simulink model "Full_load_sim_doc"  (R2020a)
settings: Solver=VariableStepAuto  StartTime=0.0  StopTime=50000  RelTol=1e-3
values from neighbouring files (symbols this model uses):
  BlySyreON = 1    [sim_starter.m]
  LiIonLilleON = 1    [sim_starter.m]
  LiIonStorON = 1    [sim_starter.m]
  LoadBlySyre = load    [sim_starter.m]
  LoadLille = load    [sim_starter.m]
  LoadLiStor = 0    [sim_starter.m]
  LoadNiMH = load    [sim_starter.m]
  LoadSaltVand = load    [sim_starter.m]
  NiMHON = 1    [sim_starter.m]
  SaltVandON = 1    [sim_starter.m]
undefined symbols (not defined in the file or in its folder): Hydride, Metal, Nickel
libraries: nesl_utility x28, fl_lib x24, powerlib x4, ee_lib x4, electricdrivelib x1
(part 2 of 2)

== system Full_load_sim_doc/Afladning/LoadSaltvandCircuit ==
  CutOff : Inport
  current : Inport  Port=2
  Constant1 : Constant  Value=0
  Controlled Current Source : fl_lib/Electrical/Electrical Sources/Controlled Current Source
  Electrical Reference1 : fl_lib/Electrical/Electrical Elements/Electrical Reference
  Gain : Gain
  Gain1 : Gain  Gain=-1
  Logical Operator1 : Logic  Operator=OR  AllPortsSameDT=off  OutDataTypeStr=boolean
  Simulink-PS Converter : nesl_utility/Simulink-PS Converter  PhysicalDomain=network_engine_domain  SubClassName=ps_input  LeftPortType=input  RightPortType=output  PseudoPeriodic=off  Frequencies=[]  NoiseDistribution=none  NoiseParameters=[]  Unit=1  AffineConversion=off  FilteringAndDerivatives=provide  SimscapeFilterOrder=1  InputFilterTimeConstant=0.001  UdotUserProvided=0
  Switch : Switch  Criteria=u2 > Threshold
  Positiv : PMIOPort  Side=Left
  Negativ : PMIOPort  Port=2  Side=Left
  wires:
  Gain/1 -> Logical Operator1/2
  Constant1/1 -> Switch/1
  Gain1/1 -> Logical Operator1/1
  CutOff/1 -> Gain1/1, Gain/1
  current/1 -> Switch/3
  Logical Operator1/1 -> Switch/2
  Switch/1 -> Simulink-PS Converter/1
  connections:
  Negativ/RConn1 -- Electrical Reference1/LConn1 -- Controlled Current Source/LConn1
  Controlled Current Source/RConn1 -- Simulink-PS Converter/RConn1
  Positiv/RConn1 -- Controlled Current Source/RConn2

== system Full_load_sim_doc/Afladning/NiMH ==
  note: Panasonic BK120AAHU
  Bus Selector : BusSelector  OutputSignals=Current (A),Voltage (V),SOC (%)
  Gain : Gain  Gain=1/100
  Ni-MH 1.2AH : electricdrivelib/Extra Sources/Battery  BatType=Nickel-Metal-Hydride  ShowTempParam=off  ThermalPreset=no  ShowAgeParam=off  NomV=1.22  NomQ=1.2  SOC=100  Batt_Tr=30  PresetModel=off  MaxQ=1.291  MinV=0.915  FullV=1.43  Dis_rate=0.240  R=0.017  Normal_OP=1.128  expZone="[1.27        0.24]"  current=[0.240 0.480 1.2]  Units=Time  Tci=20  NomT=20  T2=-30  MaxQ2=4.8  FullV2=7.1  Normal_OP2=5.655  expZone2="[6.58           1]"  Rca=0.6  ti=2000  Dp=0  Neq0=0  Tsim=1e6  Ta1=25  Qeol=5.4*0.9  Reol=0.013333*1.2  Char_age=[2.3478, 3]  Dis_age=[2.3478, 10]  N1=1500  N2=10500  N3=1000  N4=1400  Ta2=45  N5=950
  powergui : powerlib/powergui  Priority=1  SimulationMode=Continuous  SampleTime=50e-6  frequency=60  Iterations=50  frequencyindice=0  Pbase=100e6  ErrMax=1e-4  UnitsV=kV  UnitsW=MW  buscounter=0  FunctionMessages=off  echomessages=off  EnableUseOfTLC=off  CurrentSourceSwitches=off  DisableSnubberDevices=off  DisableRonSwitches=off  DisableVfSwitches=off  DisplayEquations=off  AutomaticDiscreteSolvers=off  SolverType=Tustin/Backward Euler (TBE)  Interpol=off  ExternalGateDelay=off  methode=off  Ts=100  x0status=blocks  SPID=on  SwTol=0  HookPort=off  NonlinearTolerance=1e-4  nMaxIteration=100  ContinueOnMaxIteration=off  RestoreLinks=warning  ResistiveCurrentMeasurement=off  Frange=[0:2:500]  Ylog=off  Xlog=on  ShowGrid=off  save=off  variable=ZData  structure=0  ZoomFFT=off  StartTime=0.0  cycles=1  DisplayStyle=1  fundamental=60  FreqAxis=off  MaxFrequency=1000  frequencyindicesteady=1  RmsSteady=1  display=off
  Positiv : PMIOPort  Side=Right
  Negativ : PMIOPort  Port=2  Side=Right
  VoltageLevel : Outport
  CurrentLevel : Outport  Port=2
  SOC : Outport  Port=3
  wires:
  Bus Selector/1 -> CurrentLevel/1  "<Current (A)>"
  Ni-MH 1.2AH/1 -> Bus Selector/1
  Bus Selector/2 -> VoltageLevel/1  "<Voltage (V)>"
  Bus Selector/3 -> Gain/1  "<SOC (%)>"
  Gain/1 -> SOC/1
  connections:
  Ni-MH 1.2AH/LConn1 -- Positiv/RConn1
  Ni-MH 1.2AH/LConn2 -- Negativ/RConn1

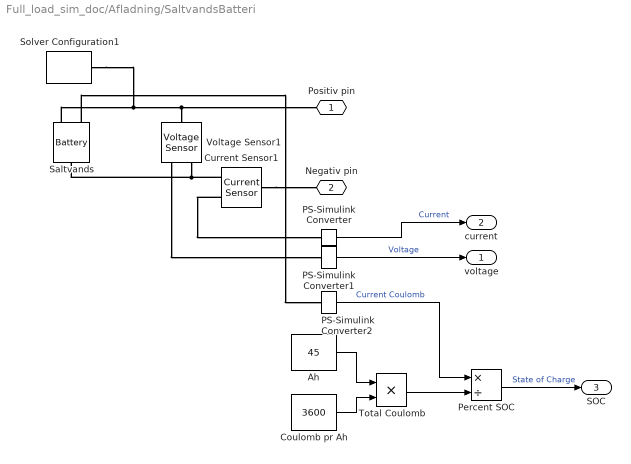
== system Full_load_sim_doc/Afladning/SaltvandsBatteri ==
  Ah : Constant  Value=45
  Coulomb pr Ah : Constant  Value=3600
  Current Sensor1 : fl_lib/Electrical/Electrical Sensors/Current Sensor
  PS-Simulink Converter : nesl_utility/PS-Simulink Converter  PhysicalDomain=network_engine_domain  SubClassName=ps_output  LeftPortType=input  RightPortType=output  PseudoPeriodic=off  Frequencies=[]  Unit=inherit  AffineConversion=off
  PS-Simulink Converter1 : nesl_utility/PS-Simulink Converter  PhysicalDomain=network_engine_domain  SubClassName=ps_output  LeftPortType=input  RightPortType=output  PseudoPeriodic=off  Frequencies=[]  Unit=inherit  AffineConversion=off
  PS-Simulink Converter2 : nesl_utility/PS-Simulink Converter  PhysicalDomain=network_engine_domain  SubClassName=ps_output  LeftPortType=input  RightPortType=output  PseudoPeriodic=off  Frequencies=[]  Unit=inherit  AffineConversion=off
  Percent SOC : Product  Inputs=*/
  Saltvands : ee_lib/Sources/Battery  Vnom=12 V  R1=0.005 Ohm  prm_AH=2  AH=45 hr*A  V1=10.8 V  AH1=2 hr*A  prm_R2=1  R2=5000 Ohm  prm_dyn=3  Rp1=0.05 Ohm  tau1=700 s  Rp2=0.01 Ohm  tau2=55 s  Rp3=0.005 Ohm  tau3=30 s  Rp4=0.005 Ohm  tau4=30 s  Rp5=0.005 Ohm  tau5=30 s  prm_fade=2  N_fade=5000  AH_fade=36 hr*A  R1_fade=2.02 Ohm  V1_fade=10.35 V  i_specify=off  i_priority=None  i=0 A  i_nominal_specify=off  i_nominal_unit=A  i_nominal_value=1  v_specify=off  v_priority=None  v=0 V  v_nominal_specify=off  v_nominal_unit=V  v_nominal_value=1  charge_specify=on  charge_priority=High  charge=45 hr*A  charge_nominal_specify=off  charge_nominal_unit=hr*A  charge_nominal_value=1  num_cycles_specify=off  num_cycles_priority=High  num_cycles=20  num_cycles_nominal_specify=off  num_cycles_nominal_unit=1  num_cycles_nominal_value=1  thermal_mass=30000 J/K  Tmeas=298.15 K  Vnom_T2=12 V  R1_T2=2.2 Ohm  V1_T2=11.4 V  R2_T2=2200 Ohm  Rp1_T2=0.005 Ohm  tau1_T2=30 s  Rp2_T2=0.005 Ohm  tau2_T2=30 s  Rp3_T2=0.005 Ohm  tau3_T2=30 s  Rp4_T2=0.005 Ohm  tau4_T2=30 s  Rp5_T2=0.005 Ohm  tau5_T2=30 s  Tmeas2=273.15 K  temperature_specify=off  temperature_priority=High  temperature=298.15 K  temperature_nominal_specify=off  temperature_nominal_unit=K  temperature_nominal_value=1
      settings: LogSimulationData=on  InternalSimscapePortConfiguration="{\"Bottom\":[],\"Left\":[{\"id\":\"p\",\"label\":\"+\",\"type\":\"foundation.electrical.electrical\"},{\"id\":\"q\",\"label\":\"q\",\"type\":\"output\"}],\"Right\":[{\"id\":\"n\",\"label\":\"-\",\"type\":\"foundation.electrical.electrical\"}],\"Top\":[]}"
  Solver Configuration1 : nesl_utility/Solver Configuration  PhysicalDomain=network_engine_domain  SubClassName=solver  LeftPortType=input  RightPortType=generic  Tones=[]  Harmonics=[]  SimulateNoise=off  Profile=off  UseLocalSampling=off  EnableSwitchedLinearOptims=on  FrequencyDomain=off  UseCCode=off  RelTol=0.001  AbsTol=1e-06  MinStep=1e-09  ToWorkspace=off  RevertToSquareIcSolve=off  NumHomotopyIterations=100  PhasorMode=off  PhasorModeNumHarmonics=1  DoDC=off  ResidualTolerance=1e-09  UseLocalSolver=off  LocalSolverChoice=NE_BACKWARD_EULER_ADVANCER  LocalSolverSampleTime=0.001  DoFixedCost=off  MaxNonlinIter=3  MaxModeIter=2  LinearAlgebra=auto  EquationFormulation=NE_TIME_EF  DelaysMemoryBudget=1024  AutomaticFiltering=on  FilteringTimeConstant=0.001  PartitionStorageMethod=AS_NEEDED  PartitionMemoryBudget=1024  PartitionMethod=ROBUST
  Total Coulomb : Product  Inputs=**
  Voltage Sensor1 : fl_lib/Electrical/Electrical Sensors/Voltage Sensor
  Positiv pin : PMIOPort  Side=Right
  Negativ pin : PMIOPort  Port=2  Side=Right
  voltage : Outport
  current : Outport  Port=2
  SOC : Outport  Port=3
  wires:
  PS-Simulink Converter/1 -> current/1  "Current"
  PS-Simulink Converter1/1 -> voltage/1  "Voltage"
  Total Coulomb/1 -> Percent SOC/2
  PS-Simulink Converter2/1 -> Percent SOC/1  "Current Coulomb"
  Percent SOC/1 -> SOC/1  "State of Charge"
  Ah/1 -> Total Coulomb/1
  Coulomb pr Ah/1 -> Total Coulomb/2
  connections:
  Voltage Sensor1/RConn2 -- Saltvands/RConn1 -- Current Sensor1/RConn2
  Saltvands/LConn1 -- Positiv pin/RConn1 -- Voltage Sensor1/LConn1 -- Solver Configuration1/RConn1
  Current Sensor1/LConn1 -- Negativ pin/RConn1
  Current Sensor1/RConn1 -- PS-Simulink Converter/LConn1
  Voltage Sensor1/RConn1 -- PS-Simulink Converter1/LConn1
  Saltvands/LConn2 -- PS-Simulink Converter2/LConn1

== stateflow chart Full_load_sim_doc/Afladning/BMS Saltvand /BMS kontrol ==
  state Idle
    %I dette stadie er vores BMS idle, da der hverken sker opladning eller afladning af vores batteri.
    entry:
    cutOff = 0;
  state Charging
    during:
    discharging = 0;
    charging = 1;
    state dischargingLevel
      entry:
      cutOff = 0;
    state currentLevel
      entry:
      cutOff = 1;
    state voltageLevel
      entry:
      cutOff = 1;
    (default) -> Charging.dischargingLevel
    Charging.dischargingLevel -> Charging.currentLevel [order 2] : [currentLevel >= currentUpperLimitCharge | SOC >= 1]{cutOff =  1;}
    Charging.currentLevel -> Charging.dischargingLevel : [currentLevel <= currentUpperLimitCharge]{cutOff = 0;}
    Charging.dischargingLevel -> Charging.voltageLevel [order 1] : [voltageLevel >= voltageUpperLimit | SOC >= 1]{cutOff = 1;}
  state Discharge
    entry:
    discharging = 1;
    charging = 0;
    state dischargingLevel
    state currentLevel
    state voltageLevel
    (default) -> Discharge.dischargingLevel
    Discharge.dischargingLevel -> Discharge.currentLevel [order 2] : [currentLevel >= currentUpperLimit | SOC <= 0.05]{cutOff =  1;}
    Discharge.currentLevel -> Discharge.dischargingLevel : [currentLevel <= currentUpperLimit]{cutOff = 0;}
    Discharge.dischargingLevel -> Discharge.voltageLevel [order 1] : [voltageLevel <= voltageLowerLimit | SOC <= 0.05]{cutOff = 1;}
  (default) -> Idle
  Discharge -> Idle [order 2] : [currentLevel == 0]
  Idle -> Discharge [order 1] : [currentLevel >= 0]
  Charging -> Idle [order 2] : [currentLevel == 0]
  Idle -> Charging [order 2] : [currentLevel <= 0 ]
  Discharge -> Charging [order 1] : [currentLevel <= 0 ]
  Charging -> Discharge [order 1] : [currentLevel >= 0]
  data: currentLevel input; voltageLevel input; discharging local; charging local; cutOff output; currentUpperLimit local =20; SOC input; voltageLowerLimit local =9.0; voltageUpperLimit local =15; currentUpperLimitCharge local =20

== stateflow chart Full_load_sim_doc/Afladning/BMS Li ion Stor/BMS kontrol ==
  state Idle
    %I dette stadie er vores BMS idle, da der hverken sker opladning eller afladning af vores batteri.
  state Charging
    during:
    discharging = 0;
    charging = 1;
    state dischargingLevel
      entry:
      cutOff = 0;
    state currentLevel
      entry:
      cutOff = 1;
    state voltageLevel
      entry:
      cutOff = 1;
    (default) -> Charging.dischargingLevel
    Charging.dischargingLevel -> Charging.currentLevel [order 2] : [currentLevel >= currentUpperLimitCharge | SOC >= 1]{cutOff =  1;}
    Charging.currentLevel -> Charging.dischargingLevel : [currentLevel <= currentUpperLimitCharge]{cutOff = 0;}
    Charging.dischargingLevel -> Charging.voltageLevel [order 1] : [voltageLevel >= voltageUpperLimit | SOC >= 1]{cutOff = 1;}
  state Discharge
    entry:
    discharging = 1;
    charging = 0;
    state dischargingLevel
    state currentLevel
    state voltageLevel
    (default) -> Discharge.dischargingLevel
    Discharge.dischargingLevel -> Discharge.currentLevel [order 2] : [currentLevel >= currentUpperLimit | SOC <= 0.05]{cutOff =  1;}
    Discharge.currentLevel -> Discharge.dischargingLevel : [currentLevel <= currentUpperLimit]{cutOff = 0;}
    Discharge.dischargingLevel -> Discharge.voltageLevel [order 1] : [voltageLevel <= voltageLowerLimit | SOC <= 0.05]{cutOff = 1;}
  (default) -> Idle
  Discharge -> Idle [order 2] : [currentLevel == 0]
  Idle -> Discharge [order 1] : [currentLevel >= 0]
  Charging -> Idle [order 2] : [currentLevel == 0]
  Idle -> Charging [order 2] : [currentLevel <= 0 ]
  Discharge -> Charging [order 1] : [currentLevel <= 0 ]
  Charging -> Discharge [order 1] : [currentLevel >= 0]
  data: currentLevel input; voltageLevel input; discharging local; charging local; cutOff output; currentUpperLimit local =20; SOC input; voltageLowerLimit local =9.0; voltageUpperLimit local =15; currentUpperLimitCharge local =20

== stateflow chart Full_load_sim_doc/Afladning/BMS Li Ion Lille/BMS kontrol ==
  state Idle
    %I dette stadie er vores BMS idle, da der hverken sker opladning eller afladning af vores batteri.
  state Charging
    during:
    discharging = 0;
    charging = 1;
    state dischargingLevel
      entry:
      cutOff = 0;
    state currentLevel
      entry:
      cutOff = 1;
    state voltageLevel
      entry:
      cutOff = 1;
    (default) -> Charging.dischargingLevel
    Charging.dischargingLevel -> Charging.currentLevel [order 2] : [currentLevel >= currentUpperLimitCharge | SOC >= 1]{cutOff =  1;}
    Charging.currentLevel -> Charging.dischargingLevel : [currentLevel <= currentUpperLimitCharge]{cutOff = 0;}
    Charging.dischargingLevel -> Charging.voltageLevel [order 1] : [voltageLevel >= voltageUpperLimit | SOC >= 1]{cutOff = 1;}
  state Discharge
    entry:
    discharging = 1;
    charging = 0;
    state dischargingLevel
    state currentLevel
    state voltageLevel
    (default) -> Discharge.dischargingLevel
    Discharge.dischargingLevel -> Discharge.currentLevel [order 2] : [currentLevel >= currentUpperLimit | SOC <= 0.05]{cutOff =  1;}
    Discharge.currentLevel -> Discharge.dischargingLevel : [currentLevel <= currentUpperLimit]{cutOff = 0;}
    Discharge.dischargingLevel -> Discharge.voltageLevel [order 1] : [voltageLevel <= voltageLowerLimit | SOC <= 0.05]{cutOff = 1;}
  (default) -> Idle
  Discharge -> Idle [order 2] : [currentLevel == 0]
  Idle -> Discharge [order 1] : [currentLevel >= 0]
  Charging -> Idle [order 2] : [currentLevel == 0]
  Idle -> Charging [order 2] : [currentLevel <= 0 ]
  Discharge -> Charging [order 1] : [currentLevel <= 0 ]
  Charging -> Discharge [order 1] : [currentLevel >= 0]
  data: currentLevel input; voltageLevel input; discharging local; charging local; cutOff output; currentUpperLimit local =0.52; SOC input; voltageLowerLimit local =3; voltageUpperLimit local =4.2; currentUpperLimitCharge local =0.52

== stateflow chart Full_load_sim_doc/Afladning/BMS NiMH/BMS kontrol ==
  state Idle
    %I dette stadie er vores BMS idle, da der hverken sker opladning eller afladning af vores batteri.
  state Charging
    during:
    discharging = 0;
    charging = 1;
    state dischargingLevel
      entry:
      cutOff = 0;
    state currentLevel
      entry:
      cutOff = 1;
    state voltageLevel
      entry:
      cutOff = 1;
    (default) -> Charging.dischargingLevel
    Charging.dischargingLevel -> Charging.currentLevel [order 2] : [currentLevel >= currentUpperLimitCharge | SOC >= 1]{cutOff =  1;}
    Charging.currentLevel -> Charging.dischargingLevel : [currentLevel <= currentUpperLimitCharge]{cutOff = 0;}
    Charging.dischargingLevel -> Charging.voltageLevel [order 1] : [voltageLevel >= voltageUpperLimit | SOC >= 1]{cutOff = 1;}
  state Discharge
    entry:
    discharging = 1;
    charging = 0;
    state dischargingLevel
    state currentLevel
    state voltageLevel
    (default) -> Discharge.dischargingLevel
    Discharge.dischargingLevel -> Discharge.currentLevel [order 2] : [currentLevel >= currentUpperLimit | SOC <=0.05]{cutOff =  1;}
    Discharge.currentLevel -> Discharge.dischargingLevel : [currentLevel <= currentUpperLimit]{cutOff = 0;}
    Discharge.dischargingLevel -> Discharge.voltageLevel [order 1] : [voltageLevel <= voltageLowerLimit | SOC <= 0.05]{cutOff = 1;}
  (default) -> Idle
  Discharge -> Idle [order 2] : [currentLevel == 0]
  Idle -> Discharge [order 1] : [currentLevel >= 0]
  Charging -> Idle [order 2] : [currentLevel == 0]
  Idle -> Charging [order 2] : [currentLevel <= 0 ]
  Discharge -> Charging [order 1] : [currentLevel <= 0 ]
  Charging -> Discharge [order 1] : [currentLevel >= 0]
  data: currentLevel input; voltageLevel input; discharging local; charging local; cutOff output; currentUpperLimit local =1.2; SOC input; voltageLowerLimit local =1; voltageUpperLimit local =1.43; currentUpperLimitCharge local =1

== stateflow chart Full_load_sim_doc/Afladning/BMS BlySyre/BMS kontrol ==
  state Idle
    %I dette stadie er vores BMS idle, da der hverken sker opladning eller afladning af vores batteri.
  state Charging
    during:
    discharging = 0;
    charging = 1;
    state dischargingLevel
      entry:
      cutOff = 0;
    state currentLevel
      entry:
      cutOff = 1;
    state voltageLevel
      entry:
      cutOff = 1;
    (default) -> Charging.dischargingLevel
    Charging.dischargingLevel -> Charging.currentLevel [order 2] : [currentLevel >= currentUpperLimitCharge | SOC >= 1]{cutOff =  1;}
    Charging.currentLevel -> Charging.dischargingLevel : [currentLevel <= currentUpperLimitCharge]{cutOff = 0;}
    Charging.dischargingLevel -> Charging.voltageLevel [order 1] : [voltageLevel >= voltageUpperLimit | SOC >= 1]{cutOff = 1;}
  state Discharge
    entry:
    discharging = 1;
    charging = 0;
    state dischargingLevel
    state currentLevel
    state voltageLevel
    (default) -> Discharge.dischargingLevel
    Discharge.dischargingLevel -> Discharge.currentLevel [order 2] : [currentLevel >= currentUpperLimit | SOC <= 0.05]{cutOff =  1;}
    Discharge.currentLevel -> Discharge.dischargingLevel : [currentLevel <= currentUpperLimit]{cutOff = 0;}
    Discharge.dischargingLevel -> Discharge.voltageLevel [order 1] : [voltageLevel <= voltageLowerLimit | SOC <= 0.05]{cutOff = 1;}
  (default) -> Idle
  Discharge -> Idle [order 2] : [currentLevel == 0]
  Idle -> Discharge [order 1] : [currentLevel >= 0]
  Charging -> Idle [order 2] : [currentLevel == 0]
  Idle -> Charging [order 2] : [currentLevel <= 0 ]
  Discharge -> Charging [order 1] : [currentLevel <= 0 ]
  Charging -> Discharge [order 1] : [currentLevel >= 0]
  data: currentLevel input; voltageLevel input; discharging local; charging local; cutOff output; currentUpperLimit local =20; SOC input; voltageLowerLimit local =10; voltageUpperLimit local =15; currentUpperLimitCharge local =20
